simulink model "c00004M_harness"  (R2018a)
settings: Solver=FixedStepAuto  StartTime=0.0  StopTime=300  FixedStep=0.1  RelTol=1e-3
undefined symbols (not defined in the file): A1, hmax, R1, R2, sigbuilder_block, TempThreshold
(part 1 of 14)
settings Model: Creator=aarrieta  LastModifiedBy=umarkiegi

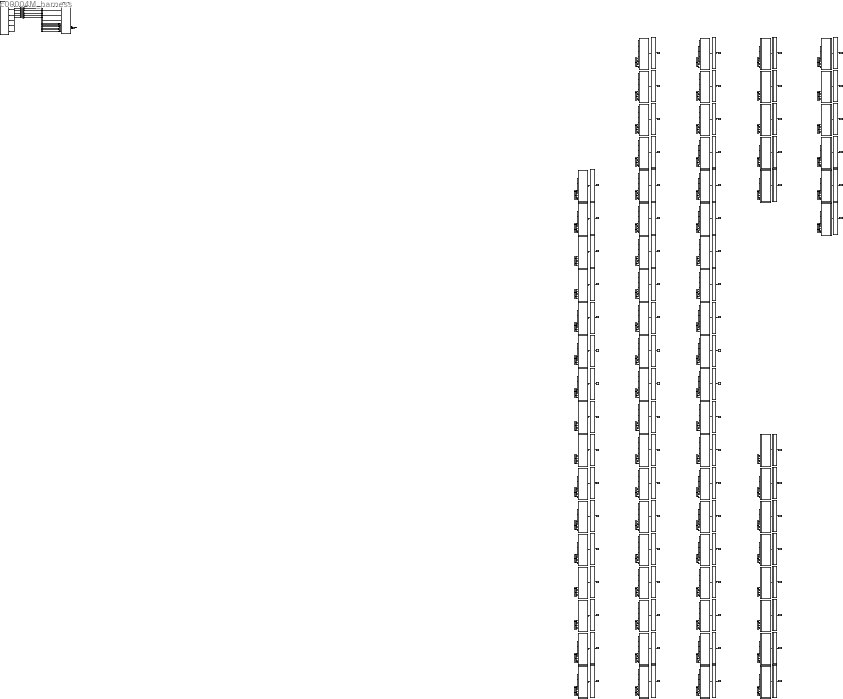
== system c00004M_harness ==
  CPSUT : Subsystem
  Eval164 : Subsystem
  Eval165 : Subsystem
  Eval166 : Subsystem
  Eval167 : Subsystem
  Eval168 : Subsystem
  Eval169 : Subsystem
  Eval170 : Subsystem
  Eval171 : Subsystem
  Eval172 : Subsystem
  Eval173 : Subsystem
  Eval174 : Subsystem
  Eval175 : Subsystem
  Eval176 : Subsystem
  Eval177 : Subsystem
  Eval178 : Subsystem
  Eval179 : Subsystem
  Eval180 : Subsystem
  Eval181 : Subsystem
  Eval182 : Subsystem
  Eval183 : Subsystem
  Eval184 : Subsystem
  Eval185 : Subsystem
  Eval186 : Subsystem
  Eval187 : Subsystem
  Eval188 : Subsystem
  Eval189 : Subsystem
  Eval190 : Subsystem
  Eval191 : Subsystem
  Eval192 : Subsystem
  Eval193 : Subsystem
  Eval194 : Subsystem
  Eval195 : Subsystem
  Eval196 : Subsystem
  Eval197 : Subsystem
  Eval198 : Subsystem
  Eval199 : Subsystem
  Eval200 : Subsystem
  Eval201 : Subsystem
  Eval202 : Subsystem
  Eval203 : Subsystem
  Eval204 : Subsystem
  Eval205 : Subsystem
  Eval206 : Subsystem
  Eval207 : Subsystem
  Eval208 : Subsystem
  Eval209 : Subsystem
  Eval210 : Subsystem
  Eval211 : Subsystem
  Eval212 : Subsystem
  Eval213 : Subsystem
  Eval214 : Subsystem
  Eval215 : Subsystem
  Eval216 : Subsystem
  Eval217 : Subsystem
  Eval218 : Subsystem
  Eval219 : Subsystem
  Eval220 : Subsystem
  Eval221 : Subsystem
  Eval222 : Subsystem
  Eval223 : Subsystem
  Eval224 : Subsystem
  Eval232 : Subsystem
  Eval233 : Subsystem
  Eval234 : Subsystem
  Eval235 : Subsystem
  Eval236 : Subsystem
  Eval237 : Subsystem
  Eval238 : Subsystem
  Eval239 : Subsystem
  Eval240 : Subsystem
  Eval241 : Subsystem
  Eval242 : Subsystem
  Eval243 : Subsystem
  Eval244 : Subsystem
  Eval245 : Subsystem
  Inputs : Subsystem  Tag=STV Subsys  LoadFcn=sigbuilder_block('load');  StartFcn=sigbuilder_block('start');  StopFcn=sigbuilder_block('stop');  ClipboardFcn=sigbuilder_block('clipboard');  mask(Sigbuilder block){tuvar=[0:10]}
      mask init:
      | if ~strcmp(get_param(bdroot(gcb),'SimulationStatus'),'stopped'),tuvar = sigbuilder_block('maskInit'); end
      settings: CopyFcn=sigbuilder_block('copy');  DeleteFcn=sigbuilder_block('delete');  ModelCloseFcn=sigbuilder_block('modelClose');  PreSaveFcn=sigbuilder_block('preSave');  PauseFcn=sigbuilder_block('pause');  ContinueFcn=sigbuilder_block('continue');  NameChangeFcn=sigbuilder_block('namechange');  OpenFcn=sigbuilder_block('open',[276.75 163.5 675.75 486.75 ]);  CloseFcn=sigbuilder_block('close');
      mask Display: plot(0, 0, 100, 100,[2, 2, 32, 32, 2], [68, 8, 8, 68, 68],[32, 2], [38, 38], [32, 19, 2],[53, 60, 44], [32, 17, 17, 2],[16, 16, 31, 31]);txt = getActiveGroup(gcbh);text(2, 100, txt,'verticalAlignment', 'top');
  M165 : Subsystem
  M166 : Subsystem
  M167 : Subsystem
  M168 : Subsystem
  M169 : Subsystem
  M170 : Subsystem
  M171 : Subsystem
  M172 : Subsystem
  M173 : Subsystem
  M174 : Subsystem
  M175 : Subsystem
  M176 : Subsystem
  M177 : Subsystem
  M178 : Subsystem
  M179 : Subsystem
  M180 : Subsystem
  M181 : Subsystem
  M182 : Subsystem
  M183 : Subsystem
  M184 : Subsystem
  M185 : Subsystem
  M186 : Subsystem
  M187 : Subsystem
  M188 : Subsystem
  M189 : Subsystem
  M190 : Subsystem
  M191 : Subsystem
  M192 : Subsystem
  M193 : Subsystem
  M194 : Subsystem
  M195 : Subsystem
  M196 : Subsystem
  M197 : Subsystem
  M198 : Subsystem
  M199 : Subsystem
  M200 : Subsystem
  M201 : Subsystem
  M202 : Subsystem
  M203 : Subsystem
  M204 : Subsystem
  M205 : Subsystem
  M206 : Subsystem
  M207 : Subsystem
  M208 : Subsystem
  M209 : Subsystem
  M210 : Subsystem
  M211 : Subsystem
  M212 : Subsystem
  M213 : Subsystem
  M214 : Subsystem
  M215 : Subsystem
  M216 : Subsystem
  M217 : Subsystem
  M218 : Subsystem
  M219 : Subsystem
  M220 : Subsystem
  M221 : Subsystem
  M222 : Subsystem
  M223 : Subsystem
  M224 : Subsystem
  M225 : Subsystem
  M233 : Subsystem
  M234 : Subsystem
  M235 : Subsystem
  M236 : Subsystem
  M237 : Subsystem
  M238 : Subsystem
  M239 : Subsystem
  M240 : Subsystem
  M241 : Subsystem
  M242 : Subsystem
  M243 : Subsystem
  M244 : Subsystem
  M245 : Subsystem
  M246 : Subsystem
  To Workspace164 : ToWorkspace  VariableName=mutant165  SampleTime=-1
  To Workspace165 : ToWorkspace  VariableName=mutant166  SampleTime=-1
  To Workspace166 : ToWorkspace  VariableName=mutant167  SampleTime=-1
  To Workspace167 : ToWorkspace  VariableName=mutant168  SampleTime=-1
  To Workspace168 : ToWorkspace  VariableName=mutant169  SampleTime=-1
  To Workspace169 : ToWorkspace  VariableName=mutant170  SampleTime=-1
  To Workspace170 : ToWorkspace  VariableName=mutant171  SampleTime=-1
  To Workspace171 : ToWorkspace  VariableName=mutant172  SampleTime=-1
  To Workspace172 : ToWorkspace  VariableName=mutant173  SampleTime=-1
  To Workspace173 : ToWorkspace  VariableName=mutant174  SampleTime=-1
  To Workspace174 : ToWorkspace  VariableName=mutant175  SampleTime=-1
  To Workspace175 : ToWorkspace  VariableName=mutant176  SampleTime=-1
  To Workspace176 : ToWorkspace  VariableName=mutant177  SampleTime=-1
  To Workspace177 : ToWorkspace  VariableName=mutant178  SampleTime=-1
  To Workspace178 : ToWorkspace  VariableName=mutant179  SampleTime=-1
  To Workspace179 : ToWorkspace  VariableName=mutant180  SampleTime=-1
  To Workspace180 : ToWorkspace  VariableName=mutant181  SampleTime=-1
  To Workspace181 : ToWorkspace  VariableName=mutant182  SampleTime=-1
  To Workspace182 : ToWorkspace  VariableName=mutant183  SampleTime=-1
  To Workspace183 : ToWorkspace  VariableName=mutant184  SampleTime=-1
  To Workspace184 : ToWorkspace  VariableName=mutant185  SampleTime=-1
  To Workspace185 : ToWorkspace  VariableName=mutant186  SampleTime=-1
  To Workspace186 : ToWorkspace  VariableName=mutant187  SampleTime=-1
  To Workspace187 : ToWorkspace  VariableName=mutant188  SampleTime=-1
  To Workspace188 : ToWorkspace  VariableName=mutant189  SampleTime=-1
  To Workspace189 : ToWorkspace  VariableName=mutant190  SampleTime=-1
  To Workspace190 : ToWorkspace  VariableName=mutant191  SampleTime=-1
  To Workspace191 : ToWorkspace  VariableName=mutant192  SampleTime=-1
  To Workspace192 : ToWorkspace  VariableName=mutant193  SampleTime=-1
  To Workspace193 : ToWorkspace  VariableName=mutant194  SampleTime=-1
  To Workspace194 : ToWorkspace  VariableName=mutant195  SampleTime=-1
  To Workspace195 : ToWorkspace  VariableName=mutant196  SampleTime=-1
  To Workspace196 : ToWorkspace  VariableName=mutant197  SampleTime=-1
  To Workspace197 : ToWorkspace  VariableName=mutant198  SampleTime=-1
  To Workspace198 : ToWorkspace  VariableName=mutant199  SampleTime=-1
  To Workspace199 : ToWorkspace  VariableName=mutant200  SampleTime=-1
  To Workspace200 : ToWorkspace  VariableName=mutant201  SampleTime=-1
  To Workspace201 : ToWorkspace  VariableName=mutant202  SampleTime=-1
  To Workspace202 : ToWorkspace  VariableName=mutant203  SampleTime=-1
  To Workspace203 : ToWorkspace  VariableName=mutant204  SampleTime=-1
  To Workspace204 : ToWorkspace  VariableName=mutant205  SampleTime=-1
  To Workspace205 : ToWorkspace  VariableName=mutant206  SampleTime=-1
  To Workspace206 : ToWorkspace  VariableName=mutant207  SampleTime=-1
  To Workspace207 : ToWorkspace  VariableName=mutant208  SampleTime=-1
  To Workspace208 : ToWorkspace  VariableName=mutant209  SampleTime=-1
  To Workspace209 : ToWorkspace  VariableName=mutant210  SampleTime=-1
  To Workspace210 : ToWorkspace  VariableName=mutant211  SampleTime=-1
  To Workspace211 : ToWorkspace  VariableName=mutant212  SampleTime=-1
  To Workspace212 : ToWorkspace  VariableName=mutant213  SampleTime=-1
  To Workspace213 : ToWorkspace  VariableName=mutant214  SampleTime=-1
  To Workspace214 : ToWorkspace  VariableName=mutant215  SampleTime=-1
  To Workspace215 : ToWorkspace  VariableName=mutant216  SampleTime=-1
  To Workspace216 : ToWorkspace  VariableName=mutant217  SampleTime=-1
  To Workspace217 : ToWorkspace  VariableName=mutant218  SampleTime=-1
  To Workspace218 : ToWorkspace  VariableName=mutant219  SampleTime=-1
  To Workspace219 : ToWorkspace  VariableName=mutant220  SampleTime=-1
  To Workspace220 : ToWorkspace  VariableName=mutant221  SampleTime=-1
  To Workspace221 : ToWorkspace  VariableName=mutant222  SampleTime=-1
  To Workspace222 : ToWorkspace  VariableName=mutant223  SampleTime=-1
  To Workspace223 : ToWorkspace  VariableName=mutant224  SampleTime=-1
  To Workspace224 : ToWorkspace  VariableName=mutant225  SampleTime=-1
  To Workspace232 : ToWorkspace  VariableName=mutant233  SampleTime=-1
  To Workspace233 : ToWorkspace  VariableName=mutant234  SampleTime=-1
  To Workspace234 : ToWorkspace  VariableName=mutant235  SampleTime=-1
  To Workspace235 : ToWorkspace  VariableName=mutant236  SampleTime=-1
  To Workspace236 : ToWorkspace  VariableName=mutant237  SampleTime=-1
  To Workspace237 : ToWorkspace  VariableName=mutant238  SampleTime=-1
  To Workspace238 : ToWorkspace  VariableName=mutant239  SampleTime=-1
  To Workspace239 : ToWorkspace  VariableName=mutant240  SampleTime=-1
  To Workspace240 : ToWorkspace  VariableName=mutant241  SampleTime=-1
  To Workspace241 : ToWorkspace  VariableName=mutant242  SampleTime=-1
  To Workspace242 : ToWorkspace  VariableName=mutant243  SampleTime=-1
  To Workspace243 : ToWorkspace  VariableName=mutant244  SampleTime=-1
  To Workspace244 : ToWorkspace  VariableName=mutant245  SampleTime=-1
  To Workspace245 : ToWorkspace  VariableName=mutant246  SampleTime=-1
  dtc_CT3 : DataTypeConversion
  dtc_E3 : DataTypeConversion
  dtc_EB3 : DataTypeConversion
  dtc_F3 : DataTypeConversion
  dtc_MR3 : DataTypeConversion
  dtc_T3 : DataTypeConversion
  LL3 : Outport
  tag scope: out3=global
  wires:
  CPSUT/1(LL3) -> [out3], LL3/1
  [in13] -> M165/1(CT3)
  [in14] -> M165/2(F3)
  [in15] -> M165/3(E3)
  [in16] -> M165/4(MR3)
  [in17] -> M165/5(T3)
  [in18] -> M165/6(EB3)
  M165/1(LL3) -> Eval164/1(In3)
  Eval164/1(Out1) -> To Workspace164/1
  [in13] -> M166/1(CT3)
  [in14] -> M166/2(F3)
  [in15] -> M166/3(E3)
  [in16] -> M166/4(MR3)
  [in17] -> M166/5(T3)
  [in18] -> M166/6(EB3)
  M166/1(LL3) -> Eval165/1(In3)
  Eval165/1(Out1) -> To Workspace165/1
  [in13] -> M167/1(CT3)
  [in14] -> M167/2(F3)
  [in15] -> M167/3(E3)
  [in16] -> M167/4(MR3)
  [in17] -> M167/5(T3)
  [in18] -> M167/6(EB3)
  M167/1(LL3) -> Eval166/1(In3)
  Eval166/1(Out1) -> To Workspace166/1
  [in13] -> M168/1(CT3)
  [in14] -> M168/2(F3)
  [in15] -> M168/3(E3)
  [in16] -> M168/4(MR3)
  [in17] -> M168/5(T3)
  [in18] -> M168/6(EB3)
  M168/1(LL3) -> Eval167/1(In3)
  Eval167/1(Out1) -> To Workspace167/1
  [in13] -> M169/1(CT3)
  [in14] -> M169/2(F3)
  [in15] -> M169/3(E3)
  [in16] -> M169/4(MR3)
  [in17] -> M169/5(T3)
  [in18] -> M169/6(EB3)
  M169/1(LL3) -> Eval168/1(In3)
  Eval168/1(Out1) -> To Workspace168/1
  [in13] -> M170/1(CT3)
  [in14] -> M170/2(F3)
  [in15] -> M170/3(E3)
  [in16] -> M170/4(MR3)
  [in17] -> M170/5(T3)
  [in18] -> M170/6(EB3)
  M170/1(LL3) -> Eval169/1(In3)
  Eval169/1(Out1) -> To Workspace169/1
  [in13] -> M171/1(CT3)
  [in14] -> M171/2(F3)
  [in15] -> M171/3(E3)
  [in16] -> M171/4(MR3)
  [in17] -> M171/5(T3)
  [in18] -> M171/6(EB3)
  M171/1(LL3) -> Eval170/1(In3)
  Eval170/1(Out1) -> To Workspace170/1
  [in13] -> M172/1(CT3)
  [in14] -> M172/2(F3)
  [in15] -> M172/3(E3)
  [in16] -> M172/4(MR3)
  [in17] -> M172/5(T3)
  [in18] -> M172/6(EB3)
  M172/1(LL3) -> Eval171/1(In3)
  Eval171/1(Out1) -> To Workspace171/1
  [in13] -> M173/1(CT3)
  [in14] -> M173/2(F3)
  [in15] -> M173/3(E3)
  [in16] -> M173/4(MR3)
  [in17] -> M173/5(T3)
  [in18] -> M173/6(EB3)
  M173/1(LL3) -> Eval172/1(In3)
  Eval172/1(Out1) -> To Workspace172/1
  [in13] -> M174/1(CT3)
  [in14] -> M174/2(F3)
  [in15] -> M174/3(E3)
  [in16] -> M174/4(MR3)
  [in17] -> M174/5(T3)
  [in18] -> M174/6(EB3)
  M174/1(LL3) -> Eval173/1(In3)
  Eval173/1(Out1) -> To Workspace173/1
  [in13] -> M175/1(CT3)
  [in14] -> M175/2(F3)
  [in15] -> M175/3(E3)
  [in16] -> M175/4(MR3)
  [in17] -> M175/5(T3)
  [in18] -> M175/6(EB3)
  M175/1(LL3) -> Eval174/1(In3)
  Eval174/1(Out1) -> To Workspace174/1
  [in13] -> M176/1(CT3)
  [in14] -> M176/2(F3)
  [in15] -> M176/3(E3)
  [in16] -> M176/4(MR3)
  [in17] -> M176/5(T3)
  [in18] -> M176/6(EB3)
  M176/1(LL3) -> Eval175/1(In3)
  Eval175/1(Out1) -> To Workspace175/1
  [in13] -> M177/1(CT3)
  [in14] -> M177/2(F3)
  [in15] -> M177/3(E3)
  [in16] -> M177/4(MR3)
  [in17] -> M177/5(T3)
  [in18] -> M177/6(EB3)
  M177/1(LL3) -> Eval176/1(In3)
  Eval176/1(Out1) -> To Workspace176/1
  [in13] -> M178/1(CT3)
  [in14] -> M178/2(F3)
  [in15] -> M178/3(E3)
  [in16] -> M178/4(MR3)
  [in17] -> M178/5(T3)
  [in18] -> M178/6(EB3)
  M178/1(LL3) -> Eval177/1(In3)
  Eval177/1(Out1) -> To Workspace177/1
  [in13] -> M179/1(CT3)
  [in14] -> M179/2(F3)
  [in15] -> M179/3(E3)
  [in16] -> M179/4(MR3)
  [in17] -> M179/5(T3)
  [in18] -> M179/6(EB3)
  M179/1(LL3) -> Eval178/1(In3)
  Eval178/1(Out1) -> To Workspace178/1
  [in13] -> M180/1(CT3)
  [in14] -> M180/2(F3)
  [in15] -> M180/3(E3)
  [in16] -> M180/4(MR3)
  [in17] -> M180/5(T3)
  [in18] -> M180/6(EB3)
  M180/1(LL3) -> Eval179/1(In3)
  Eval179/1(Out1) -> To Workspace179/1
  [in13] -> M181/1(CT3)
  [in14] -> M181/2(F3)
  [in15] -> M181/3(E3)
  [in16] -> M181/4(MR3)
  [in17] -> M181/5(T3)
  [in18] -> M181/6(EB3)
  M181/1(LL3) -> Eval180/1(In3)
  Eval180/1(Out1) -> To Workspace180/1
  [in13] -> M182/1(CT3)
  [in14] -> M182/2(F3)
  [in15] -> M182/3(E3)
  [in16] -> M182/4(MR3)
  [in17] -> M182/5(T3)
  [in18] -> M182/6(EB3)
  M182/1(LL3) -> Eval181/1(In3)
  Eval181/1(Out1) -> To Workspace181/1
  [in13] -> M183/1(CT3)
  [in14] -> M183/2(F3)
  [in15] -> M183/3(E3)
  [in16] -> M183/4(MR3)
  [in17] -> M183/5(T3)
  [in18] -> M183/6(EB3)
  M183/1(LL3) -> Eval182/1(In3)
  Eval182/1(Out1) -> To Workspace182/1
  [in13] -> M184/1(CT3)
  [in14] -> M184/2(F3)
  [in15] -> M184/3(E3)
  [in16] -> M184/4(MR3)
  [in17] -> M184/5(T3)
  [in18] -> M184/6(EB3)
  M184/1(LL3) -> Eval183/1(In3)
  Eval183/1(Out1) -> To Workspace183/1
  [in13] -> M185/1(CT3)
  [in14] -> M185/2(F3)
  [in15] -> M185/3(E3)
  [in16] -> M185/4(MR3)
  [in17] -> M185/5(T3)
  [in18] -> M185/6(EB3)
  M185/1(LL3) -> Eval184/1(In3)
  Eval184/1(Out1) -> To Workspace184/1
  [in13] -> M186/1(CT3)
  [in14] -> M186/2(F3)
  [in15] -> M186/3(E3)
  [in16] -> M186/4(MR3)
  [in17] -> M186/5(T3)
  [in18] -> M186/6(EB3)
  M186/1(LL3) -> Eval185/1(In3)
  Eval185/1(Out1) -> To Workspace185/1
  [in13] -> M187/1(CT3)
  [in14] -> M187/2(F3)
  [in15] -> M187/3(E3)
  [in16] -> M187/4(MR3)
  [in17] -> M187/5(T3)
  [in18] -> M187/6(EB3)
  M187/1(LL3) -> Eval186/1(In3)
  Eval186/1(Out1) -> To Workspace186/1
  [in13] -> M188/1(CT3)
  [in14] -> M188/2(F3)
  [in15] -> M188/3(E3)
  [in16] -> M188/4(MR3)
  [in17] -> M188/5(T3)
  [in18] -> M188/6(EB3)
  M188/1(LL3) -> Eval187/1(In3)
  Eval187/1(Out1) -> To Workspace187/1
  [in13] -> M189/1(CT3)
  [in14] -> M189/2(F3)
  [in15] -> M189/3(E3)
  [in16] -> M189/4(MR3)
  [in17] -> M189/5(T3)
  [in18] -> M189/6(EB3)
  M189/1(LL3) -> Eval188/1(In3)
  Eval188/1(Out1) -> To Workspace188/1
  [in13] -> M190/1(CT3)
  [in14] -> M190/2(F3)
  [in15] -> M190/3(E3)
  [in16] -> M190/4(MR3)
  [in17] -> M190/5(T3)
  [in18] -> M190/6(EB3)
  M190/1(LL3) -> Eval189/1(In3)
  Eval189/1(Out1) -> To Workspace189/1
  [in13] -> M191/1(CT3)
  [in14] -> M191/2(F3)
  [in15] -> M191/3(E3)
  [in16] -> M191/4(MR3)
  [in17] -> M191/5(T3)
  [in18] -> M191/6(EB3)
  M191/1(LL3) -> Eval190/1(In3)
  Eval190/1(Out1) -> To Workspace190/1
  [in13] -> M192/1(CT3)
  [in14] -> M192/2(F3)
  [in15] -> M192/3(E3)
  [in16] -> M192/4(MR3)
  [in17] -> M192/5(T3)
  [in18] -> M192/6(EB3)
  M192/1(LL3) -> Eval191/1(In3)
  Eval191/1(Out1) -> To Workspace191/1
  [in13] -> M193/1(CT3)
  [in14] -> M193/2(F3)
  [in15] -> M193/3(E3)
  [in16] -> M193/4(MR3)
  [in17] -> M193/5(T3)
  [in18] -> M193/6(EB3)
  M193/1(LL3) -> Eval192/1(In3)
  Eval192/1(Out1) -> To Workspace192/1
  [in13] -> M194/1(CT3)
  [in14] -> M194/2(F3)
  [in15] -> M194/3(E3)
  [in16] -> M194/4(MR3)
  [in17] -> M194/5(T3)
  [in18] -> M194/6(EB3)
  M194/1(LL3) -> Eval193/1(In3)
  Eval193/1(Out1) -> To Workspace193/1
  [in13] -> M195/1(CT3)
  [in14] -> M195/2(F3)
  [in15] -> M195/3(E3)
  [in16] -> M195/4(MR3)
  [in17] -> M195/5(T3)
  [in18] -> M195/6(EB3)
  M195/1(LL3) -> Eval194/1(In3)
  Eval194/1(Out1) -> To Workspace194/1
  [in13] -> M196/1(CT3)
  [in14] -> M196/2(F3)
  [in15] -> M196/3(E3)
  [in16] -> M196/4(MR3)
  [in17] -> M196/5(T3)
  [in18] -> M196/6(EB3)
  M196/1(LL3) -> Eval195/1(In3)
  Eval195/1(Out1) -> To Workspace195/1
  [in13] -> M197/1(CT3)
  [in14] -> M197/2(F3)
  [in15] -> M197/3(E3)
  [in16] -> M197/4(MR3)
  [in17] -> M197/5(T3)
  [in18] -> M197/6(EB3)
  M197/1(LL3) -> Eval196/1(In3)
  Eval196/1(Out1) -> To Workspace196/1
  [in13] -> M198/1(CT3)
  [in14] -> M198/2(F3)
  [in15] -> M198/3(E3)
  [in16] -> M198/4(MR3)
  [in17] -> M198/5(T3)
  [in18] -> M198/6(EB3)
  M198/1(LL3) -> Eval197/1(In3)
  Eval197/1(Out1) -> To Workspace197/1
  [in13] -> M199/1(CT3)
  [in14] -> M199/2(F3)
  [in15] -> M199/3(E3)
  [in16] -> M199/4(MR3)
  [in17] -> M199/5(T3)
  [in18] -> M199/6(EB3)
  M199/1(LL3) -> Eval198/1(In3)
  Eval198/1(Out1) -> To Workspace198/1
  [in13] -> M200/1(CT3)
  [in14] -> M200/2(F3)
  [in15] -> M200/3(E3)
  [in16] -> M200/4(MR3)
  [in17] -> M200/5(T3)
  [in18] -> M200/6(EB3)
  M200/1(LL3) -> Eval199/1(In3)
  Eval199/1(Out1) -> To Workspace199/1
  [in13] -> M201/1(CT3)
  [in14] -> M201/2(F3)
  [in15] -> M201/3(E3)
  [in16] -> M201/4(MR3)
  [in17] -> M201/5(T3)
  [in18] -> M201/6(EB3)
  M201/1(LL3) -> Eval200/1(In3)
  Eval200/1(Out1) -> To Workspace200/1
  [in13] -> M202/1(CT3)
  [in14] -> M202/2(F3)
  [in15] -> M202/3(E3)
  [in16] -> M202/4(MR3)
  [in17] -> M202/5(T3)
  [in18] -> M202/6(EB3)
  M202/1(LL3) -> Eval201/1(In3)
  Eval201/1(Out1) -> To Workspace201/1
  [in13] -> M203/1(CT3)
  [in14] -> M203/2(F3)
  [in15] -> M203/3(E3)
  [in16] -> M203/4(MR3)
  [in17] -> M203/5(T3)
  [in18] -> M203/6(EB3)
  M203/1(LL3) -> Eval202/1(In3)
  Eval202/1(Out1) -> To Workspace202/1
  [in13] -> M204/1(CT3)
  [in14] -> M204/2(F3)
  [in15] -> M204/3(E3)
  [in16] -> M204/4(MR3)
  [in17] -> M204/5(T3)
  [in18] -> M204/6(EB3)
  M204/1(LL3) -> Eval203/1(In3)
  Eval203/1(Out1) -> To Workspace203/1
  [in13] -> M205/1(CT3)
  [in14] -> M205/2(F3)
  [in15] -> M205/3(E3)
  [in16] -> M205/4(MR3)
  [in17] -> M205/5(T3)
  [in18] -> M205/6(EB3)
  M205/1(LL3) -> Eval204/1(In3)
  Eval204/1(Out1) -> To Workspace204/1
  [in13] -> M206/1(CT3)
  [in14] -> M206/2(F3)
  [in15] -> M206/3(E3)
  [in16] -> M206/4(MR3)
  [in17] -> M206/5(T3)
  [in18] -> M206/6(EB3)
  M206/1(LL3) -> Eval205/1(In3)
  Eval205/1(Out1) -> To Workspace205/1
  [in13] -> M207/1(CT3)
  [in14] -> M207/2(F3)
  [in15] -> M207/3(E3)
  [in16] -> M207/4(MR3)
  [in17] -> M207/5(T3)
  [in18] -> M207/6(EB3)
  M207/1(LL3) -> Eval206/1(In3)
  Eval206/1(Out1) -> To Workspace206/1
  [in13] -> M208/1(CT3)
  [in14] -> M208/2(F3)
  [in15] -> M208/3(E3)
  [in16] -> M208/4(MR3)
  [in17] -> M208/5(T3)
  [in18] -> M208/6(EB3)
  M208/1(LL3) -> Eval207/1(In3)
  Eval207/1(Out1) -> To Workspace207/1
  [in13] -> M209/1(CT3)
  [in14] -> M209/2(F3)
  [in15] -> M209/3(E3)
  [in16] -> M209/4(MR3)
  [in17] -> M209/5(T3)
  [in18] -> M209/6(EB3)
  M209/1(LL3) -> Eval208/1(In3)
  Eval208/1(Out1) -> To Workspace208/1
  [in13] -> M210/1(CT3)
  [in14] -> M210/2(F3)
  [in15] -> M210/3(E3)
  [in16] -> M210/4(MR3)
  [in17] -> M210/5(T3)
  [in18] -> M210/6(EB3)
  M210/1(LL3) -> Eval209/1(In3)
  Eval209/1(Out1) -> To Workspace209/1
  [in13] -> M211/1(CT3)
  [in14] -> M211/2(F3)
  [in15] -> M211/3(E3)
  [in16] -> M211/4(MR3)
  [in17] -> M211/5(T3)
  [in18] -> M211/6(EB3)
  M211/1(LL3) -> Eval210/1(In3)
  Eval210/1(Out1) -> To Workspace210/1
  [in13] -> M212/1(CT3)
  [in14] -> M212/2(F3)
  [in15] -> M212/3(E3)
  [in16] -> M212/4(MR3)
  [in17] -> M212/5(T3)
  [in18] -> M212/6(EB3)
  M212/1(LL3) -> Eval211/1(In3)
  Eval211/1(Out1) -> To Workspace211/1
  [in13] -> M213/1(CT3)
  [in14] -> M213/2(F3)
  [in15] -> M213/3(E3)
  [in16] -> M213/4(MR3)
  [in17] -> M213/5(T3)
  [in18] -> M213/6(EB3)
  M213/1(LL3) -> Eval212/1(In3)
  Eval212/1(Out1) -> To Workspace212/1
  [in13] -> M214/1(CT3)
  [in14] -> M214/2(F3)
  [in15] -> M214/3(E3)
  [in16] -> M214/4(MR3)
  [in17] -> M214/5(T3)
  [in18] -> M214/6(EB3)
  M214/1(LL3) -> Eval213/1(In3)
  Eval213/1(Out1) -> To Workspace213/1
  [in13] -> M215/1(CT3)
  [in14] -> M215/2(F3)
  [in15] -> M215/3(E3)
  [in16] -> M215/4(MR3)
  [in17] -> M215/5(T3)
  [in18] -> M215/6(EB3)
  M215/1(LL3) -> Eval214/1(In3)
  Eval214/1(Out1) -> To Workspace214/1
  [in13] -> M216/1(CT3)
  [in14] -> M216/2(F3)
  [in15] -> M216/3(E3)
  [in16] -> M216/4(MR3)
  [in17] -> M216/5(T3)
  [in18] -> M216/6(EB3)
  M216/1(LL3) -> Eval215/1(In3)
  Eval215/1(Out1) -> To Workspace215/1
  [in13] -> M217/1(CT3)
  [in14] -> M217/2(F3)
  [in15] -> M217/3(E3)
  [in16] -> M217/4(MR3)
  [in17] -> M217/5(T3)
  [in18] -> M217/6(EB3)
  M217/1(LL3) -> Eval216/1(In3)
  Eval216/1(Out1) -> To Workspace216/1
  [in13] -> M218/1(CT3)
  [in14] -> M218/2(F3)
  [in15] -> M218/3(E3)
  [in16] -> M218/4(MR3)
  [in17] -> M218/5(T3)
  [in18] -> M218/6(EB3)
  M218/1(LL3) -> Eval217/1(In3)
  Eval217/1(Out1) -> To Workspace217/1
  [in13] -> M219/1(CT3)
  [in14] -> M219/2(F3)
  [in15] -> M219/3(E3)
  [in16] -> M219/4(MR3)
  [in17] -> M219/5(T3)
  [in18] -> M219/6(EB3)
  M219/1(LL3) -> Eval218/1(In3)
  Eval218/1(Out1) -> To Workspace218/1
  [in13] -> M220/1(CT3)
  [in14] -> M220/2(F3)
  [in15] -> M220/3(E3)
  [in16] -> M220/4(MR3)
  [in17] -> M220/5(T3)
  [in18] -> M220/6(EB3)
  M220/1(LL3) -> Eval219/1(In3)
  Eval219/1(Out1) -> To Workspace219/1
  [in13] -> M221/1(CT3)
  [in14] -> M221/2(F3)
  [in15] -> M221/3(E3)
  [in16] -> M221/4(MR3)
  [in17] -> M221/5(T3)
  [in18] -> M221/6(EB3)
  M221/1(LL3) -> Eval220/1(In3)
  Eval220/1(Out1) -> To Workspace220/1
  [in13] -> M222/1(CT3)
  [in14] -> M222/2(F3)
  [in15] -> M222/3(E3)
  [in16] -> M222/4(MR3)
  [in17] -> M222/5(T3)
  [in18] -> M222/6(EB3)
  M222/1(LL3) -> Eval221/1(In3)
  Eval221/1(Out1) -> To Workspace221/1
  [in13] -> M223/1(CT3)
  [in14] -> M223/2(F3)
  [in15] -> M223/3(E3)
  [in16] -> M223/4(MR3)
  [in17] -> M223/5(T3)
  [in18] -> M223/6(EB3)
  M223/1(LL3) -> Eval222/1(In3)
  Eval222/1(Out1) -> To Workspace222/1
  [in13] -> M224/1(CT3)
  [in14] -> M224/2(F3)
  [in15] -> M224/3(E3)
  [in16] -> M224/4(MR3)
  [in17] -> M224/5(T3)
  [in18] -> M224/6(EB3)
  M224/1(LL3) -> Eval223/1(In3)
  Eval223/1(Out1) -> To Workspace223/1
  [in13] -> M225/1(CT3)
  [in14] -> M225/2(F3)
  [in15] -> M225/3(E3)
  [in16] -> M225/4(MR3)
  [in17] -> M225/5(T3)
  [in18] -> M225/6(EB3)
  M225/1(LL3) -> Eval224/1(In3)
  Eval224/1(Out1) -> To Workspace224/1
  [in13] -> M233/1(CT3)
  [in14] -> M233/2(F3)
  [in15] -> M233/3(E3)
  [in16] -> M233/4(MR3)
  [in17] -> M233/5(T3)
  [in18] -> M233/6(EB3)
  M233/1(LL3) -> Eval232/1(In3)
  Eval232/1(Out1) -> To Workspace232/1
  [in13] -> M234/1(CT3)
  [in14] -> M234/2(F3)
  [in15] -> M234/3(E3)
  [in16] -> M234/4(MR3)
  [in17] -> M234/5(T3)
  [in18] -> M234/6(EB3)
  M234/1(LL3) -> Eval233/1(In3)
  Eval233/1(Out1) -> To Workspace233/1
  [in13] -> M235/1(CT3)
  [in14] -> M235/2(F3)
  [in15] -> M235/3(E3)
  [in16] -> M235/4(MR3)
  [in17] -> M235/5(T3)
  [in18] -> M235/6(EB3)
  M235/1(LL3) -> Eval234/1(In3)
  Eval234/1(Out1) -> To Workspace234/1
  [in13] -> M236/1(CT3)
  [in14] -> M236/2(F3)
  [in15] -> M236/3(E3)
  [in16] -> M236/4(MR3)
  [in17] -> M236/5(T3)
  [in18] -> M236/6(EB3)
  M236/1(LL3) -> Eval235/1(In3)
  Eval235/1(Out1) -> To Workspace235/1
  [in13] -> M237/1(CT3)
  [in14] -> M237/2(F3)
  [in15] -> M237/3(E3)
  [in16] -> M237/4(MR3)
  [in17] -> M237/5(T3)
  [in18] -> M237/6(EB3)
  M237/1(LL3) -> Eval236/1(In3)
  Eval236/1(Out1) -> To Workspace236/1
  [in13] -> M238/1(CT3)
  [in14] -> M238/2(F3)
  [in15] -> M238/3(E3)
  [in16] -> M238/4(MR3)
  [in17] -> M238/5(T3)
  [in18] -> M238/6(EB3)
  M238/1(LL3) -> Eval237/1(In3)
  Eval237/1(Out1) -> To Workspace237/1
  [in13] -> M239/1(CT3)
  [in14] -> M239/2(F3)
  [in15] -> M239/3(E3)
  [in16] -> M239/4(MR3)
  [in17] -> M239/5(T3)
  [in18] -> M239/6(EB3)
  M239/1(LL3) -> Eval238/1(In3)
  Eval238/1(Out1) -> To Workspace238/1
  [in13] -> M240/1(CT3)
  [in14] -> M240/2(F3)
  [in15] -> M240/3(E3)
  [in16] -> M240/4(MR3)
  [in17] -> M240/5(T3)
  [in18] -> M240/6(EB3)
  M240/1(LL3) -> Eval239/1(In3)
  Eval239/1(Out1) -> To Workspace239/1
  [in13] -> M241/1(CT3)
  [in14] -> M241/2(F3)
  [in15] -> M241/3(E3)
  [in16] -> M241/4(MR3)
  [in17] -> M241/5(T3)
  [in18] -> M241/6(EB3)
  M241/1(LL3) -> Eval240/1(In3)
  Eval240/1(Out1) -> To Workspace240/1
  [in13] -> M242/1(CT3)
  [in14] -> M242/2(F3)
  [in15] -> M242/3(E3)
  [in16] -> M242/4(MR3)
  [in17] -> M242/5(T3)
  [in18] -> M242/6(EB3)
  M242/1(LL3) -> Eval241/1(In3)
  Eval241/1(Out1) -> To Workspace241/1
  [in13] -> M243/1(CT3)
  [in14] -> M243/2(F3)
  [in15] -> M243/3(E3)
  [in16] -> M243/4(MR3)
  [in17] -> M243/5(T3)
  [in18] -> M243/6(EB3)
  M243/1(LL3) -> Eval242/1(In3)
  Eval242/1(Out1) -> To Workspace242/1
  [in13] -> M244/1(CT3)
  [in14] -> M244/2(F3)
  [in15] -> M244/3(E3)
  [in16] -> M244/4(MR3)
  [in17] -> M244/5(T3)
  [in18] -> M244/6(EB3)
  M244/1(LL3) -> Eval243/1(In3)
  Eval243/1(Out1) -> To Workspace243/1
  [in13] -> M245/1(CT3)
  [in14] -> M245/2(F3)
  [in15] -> M245/3(E3)
  [in16] -> M245/4(MR3)
  [in17] -> M245/5(T3)
  [in18] -> M245/6(EB3)
  M245/1(LL3) -> Eval244/1(In3)
  Eval244/1(Out1) -> To Workspace244/1
  [in13] -> M246/1(CT3)
  [in14] -> M246/2(F3)
  [in15] -> M246/3(E3)
  [in16] -> M246/4(MR3)
  [in17] -> M246/5(T3)
  [in18] -> M246/6(EB3)
  M246/1(LL3) -> Eval245/1(In3)
  Eval245/1(Out1) -> To Workspace245/1
  Inputs/1(CT3) -> dtc_CT3/1
  dtc_CT3/1 -> CPSUT/1(CT3), [in13]
  Inputs/2(F3) -> dtc_F3/1
  dtc_F3/1 -> CPSUT/2(F3), [in14]
  Inputs/3(E3) -> dtc_E3/1
  dtc_E3/1 -> CPSUT/3(E3), [in15]
  Inputs/4(MR3) -> dtc_MR3/1
  dtc_MR3/1 -> CPSUT/4(MR3), [in16]
  Inputs/5(T3) -> dtc_T3/1
  dtc_T3/1 -> CPSUT/5(T3), [in17]
  Inputs/6(EB3) -> dtc_EB3/1
  dtc_EB3/1 -> CPSUT/6(EB3), [in18]

== system c00004M_harness/CPSUT ==
  note: VALUES
      | ---------------------------------
      | ControlType = 1 | 2 | 3
      | FillTank = 0 | 1
      | EmptyTank = 0 | 1
      | ManualReference between 0 and 1
      | Tempreature between 0 and 100
      | EmergencyButton = 0 | 1
      | LiquidLevel between 0 and 1 (hmax)
  note: Inputs For Tank2
  note: NAMES
      | --------------------------------------------
      | CT1 = ControlType Tank 1
      | F1 = Fill Tank 1
      | E1 = Empty Tank 1
      | MR1 = Manual Reference Tank1
      | T1 = Temperature Tank 1
      | EB1 = Emergency Button Tank 1
      | LL1 = Liquid Level 1
  note: Inputs For Tank3
  note: Inputs For Tank1
  CT3 : Inport
  F3 : Inport  Port=2
  E3 : Inport  Port=3
  MR3 : Inport  Port=4
  T3 : Inport  Port=5
  EB3 : Inport  Port=6
  Tank3 : Subsystem
  LL3 : Outport
  wires:
  Tank3/1(LL3) -> LL3/1
  MR3/1 -> Tank3/4(MR3)
  E3/1 -> Tank3/3(E3)
  CT3/1 -> Tank3/1(CT3)
  F3/1 -> Tank3/2(F3)
  EB3/1 -> Tank3/6(EB3)
  T3/1 -> Tank3/5(T3)

== system c00004M_harness/Eval164 ==
  In3 : Inport
  Constant1 : Constant
  Constant2 : Constant
  Data Type Conversion2 : DataTypeConversion
  Memory3 : Memory  InitialCondition=1
  MinMax : MinMax  Inputs=3
  MinMax3 : MinMax  Inputs=2
  ROOut3 : RelationalOperator  Operator===  OutDataTypeStr=boolean  RndMeth=Simplest
  Out1 : Outport
  wires:
  Data Type Conversion2/1 -> MinMax3/1
  Memory3/1 -> MinMax3/2
  ROOut3/1 -> Data Type Conversion2/1
  MinMax3/1 -> Memory3/1, MinMax/3
  In3/1 -> ROOut3/1
  [out3] -> ROOut3/2
  MinMax/1 -> Out1/1
  Constant1/1 -> MinMax/1
  Constant2/1 -> MinMax/2

== system c00004M_harness/Eval165 ==
  In3 : Inport
  Constant1 : Constant
  Constant2 : Constant
  Data Type Conversion2 : DataTypeConversion
  Memory3 : Memory  InitialCondition=1
  MinMax : MinMax  Inputs=3
  MinMax3 : MinMax  Inputs=2
  ROOut3 : RelationalOperator  Operator===  OutDataTypeStr=boolean  RndMeth=Simplest
  Out1 : Outport
  wires:
  Data Type Conversion2/1 -> MinMax3/1
  Memory3/1 -> MinMax3/2
  ROOut3/1 -> Data Type Conversion2/1
  MinMax3/1 -> Memory3/1, MinMax/3
  In3/1 -> ROOut3/1
  [out3] -> ROOut3/2
  MinMax/1 -> Out1/1
  Constant1/1 -> MinMax/1
  Constant2/1 -> MinMax/2

== system c00004M_harness/Eval166 ==
  In3 : Inport
  Constant1 : Constant
  Constant2 : Constant
  Data Type Conversion2 : DataTypeConversion
  Memory3 : Memory  InitialCondition=1
  MinMax : MinMax  Inputs=3
  MinMax3 : MinMax  Inputs=2
  ROOut3 : RelationalOperator  Operator===  OutDataTypeStr=boolean  RndMeth=Simplest
  Out1 : Outport
  wires:
  Data Type Conversion2/1 -> MinMax3/1
  Memory3/1 -> MinMax3/2
  ROOut3/1 -> Data Type Conversion2/1
  MinMax3/1 -> Memory3/1, MinMax/3
  In3/1 -> ROOut3/1
  [out3] -> ROOut3/2
  MinMax/1 -> Out1/1
  Constant1/1 -> MinMax/1
  Constant2/1 -> MinMax/2

== system c00004M_harness/Eval167 ==
  In3 : Inport
  Constant1 : Constant
  Constant2 : Constant
  Data Type Conversion2 : DataTypeConversion
  Memory3 : Memory  InitialCondition=1
  MinMax : MinMax  Inputs=3
  MinMax3 : MinMax  Inputs=2
  ROOut3 : RelationalOperator  Operator===  OutDataTypeStr=boolean  RndMeth=Simplest
  Out1 : Outport
  wires:
  Data Type Conversion2/1 -> MinMax3/1
  Memory3/1 -> MinMax3/2
  ROOut3/1 -> Data Type Conversion2/1
  MinMax3/1 -> Memory3/1, MinMax/3
  In3/1 -> ROOut3/1
  [out3] -> ROOut3/2
  MinMax/1 -> Out1/1
  Constant1/1 -> MinMax/1
  Constant2/1 -> MinMax/2

== system c00004M_harness/Eval168 ==
  In3 : Inport
  Constant1 : Constant
  Constant2 : Constant
  Data Type Conversion2 : DataTypeConversion
  Memory3 : Memory  InitialCondition=1
  MinMax : MinMax  Inputs=3
  MinMax3 : MinMax  Inputs=2
  ROOut3 : RelationalOperator  Operator===  OutDataTypeStr=boolean  RndMeth=Simplest
  Out1 : Outport
  wires:
  Data Type Conversion2/1 -> MinMax3/1
  Memory3/1 -> MinMax3/2
  ROOut3/1 -> Data Type Conversion2/1
  MinMax3/1 -> Memory3/1, MinMax/3
  In3/1 -> ROOut3/1
  [out3] -> ROOut3/2
  MinMax/1 -> Out1/1
  Constant1/1 -> MinMax/1
  Constant2/1 -> MinMax/2

== system c00004M_harness/Eval169 ==
  In3 : Inport
  Constant1 : Constant
  Constant2 : Constant
  Data Type Conversion2 : DataTypeConversion
  Memory3 : Memory  InitialCondition=1
  MinMax : MinMax  Inputs=3
  MinMax3 : MinMax  Inputs=2
  ROOut3 : RelationalOperator  Operator===  OutDataTypeStr=boolean  RndMeth=Simplest
  Out1 : Outport
  wires:
  Data Type Conversion2/1 -> MinMax3/1
  Memory3/1 -> MinMax3/2
  ROOut3/1 -> Data Type Conversion2/1
  MinMax3/1 -> Memory3/1, MinMax/3
  In3/1 -> ROOut3/1
  [out3] -> ROOut3/2
  MinMax/1 -> Out1/1
  Constant1/1 -> MinMax/1
  Constant2/1 -> MinMax/2

== system c00004M_harness/Eval170 ==
  In3 : Inport
  Constant1 : Constant
  Constant2 : Constant
  Data Type Conversion2 : DataTypeConversion
  Memory3 : Memory  InitialCondition=1
  MinMax : MinMax  Inputs=3
  MinMax3 : MinMax  Inputs=2
  ROOut3 : RelationalOperator  Operator===  OutDataTypeStr=boolean  RndMeth=Simplest
  Out1 : Outport
  wires:
  Data Type Conversion2/1 -> MinMax3/1
  Memory3/1 -> MinMax3/2
  ROOut3/1 -> Data Type Conversion2/1
  MinMax3/1 -> Memory3/1, MinMax/3
  In3/1 -> ROOut3/1
  [out3] -> ROOut3/2
  MinMax/1 -> Out1/1
  Constant1/1 -> MinMax/1
  Constant2/1 -> MinMax/2

== system c00004M_harness/Eval171 ==
  In3 : Inport
  Constant1 : Constant
  Constant2 : Constant
  Data Type Conversion2 : DataTypeConversion
  Memory3 : Memory  InitialCondition=1
  MinMax : MinMax  Inputs=3
  MinMax3 : MinMax  Inputs=2
  ROOut3 : RelationalOperator  Operator===  OutDataTypeStr=boolean  RndMeth=Simplest
  Out1 : Outport
  wires:
  Data Type Conversion2/1 -> MinMax3/1
  Memory3/1 -> MinMax3/2
  ROOut3/1 -> Data Type Conversion2/1
  MinMax3/1 -> Memory3/1, MinMax/3
  In3/1 -> ROOut3/1
  [out3] -> ROOut3/2
  MinMax/1 -> Out1/1
  Constant1/1 -> MinMax/1
  Constant2/1 -> MinMax/2

== system c00004M_harness/Eval172 ==
  In3 : Inport
  Constant1 : Constant
  Constant2 : Constant
  Data Type Conversion2 : DataTypeConversion
  Memory3 : Memory  InitialCondition=1
  MinMax : MinMax  Inputs=3
  MinMax3 : MinMax  Inputs=2
  ROOut3 : RelationalOperator  Operator===  OutDataTypeStr=boolean  RndMeth=Simplest
  Out1 : Outport
  wires:
  Data Type Conversion2/1 -> MinMax3/1
  Memory3/1 -> MinMax3/2
  ROOut3/1 -> Data Type Conversion2/1
  MinMax3/1 -> Memory3/1, MinMax/3
  In3/1 -> ROOut3/1
  [out3] -> ROOut3/2
  MinMax/1 -> Out1/1
  Constant1/1 -> MinMax/1
  Constant2/1 -> MinMax/2

== system c00004M_harness/Eval173 ==
  In3 : Inport
  Constant1 : Constant
  Constant2 : Constant
  Data Type Conversion2 : DataTypeConversion
  Memory3 : Memory  InitialCondition=1
  MinMax : MinMax  Inputs=3
  MinMax3 : MinMax  Inputs=2
  ROOut3 : RelationalOperator  Operator===  OutDataTypeStr=boolean  RndMeth=Simplest
  Out1 : Outport
  wires:
  Data Type Conversion2/1 -> MinMax3/1
  Memory3/1 -> MinMax3/2
  ROOut3/1 -> Data Type Conversion2/1
  MinMax3/1 -> Memory3/1, MinMax/3
  In3/1 -> ROOut3/1
  [out3] -> ROOut3/2
  MinMax/1 -> Out1/1
  Constant1/1 -> MinMax/1
  Constant2/1 -> MinMax/2

== system c00004M_harness/Eval174 ==
  In3 : Inport
  Constant1 : Constant
  Constant2 : Constant
  Data Type Conversion2 : DataTypeConversion
  Memory3 : Memory  InitialCondition=1
  MinMax : MinMax  Inputs=3
  MinMax3 : MinMax  Inputs=2
  ROOut3 : RelationalOperator  Operator===  OutDataTypeStr=boolean  RndMeth=Simplest
  Out1 : Outport
  wires:
  Data Type Conversion2/1 -> MinMax3/1
  Memory3/1 -> MinMax3/2
  ROOut3/1 -> Data Type Conversion2/1
  MinMax3/1 -> Memory3/1, MinMax/3
  In3/1 -> ROOut3/1
  [out3] -> ROOut3/2
  MinMax/1 -> Out1/1
  Constant1/1 -> MinMax/1
  Constant2/1 -> MinMax/2

== system c00004M_harness/Eval175 ==
  In3 : Inport
  Constant1 : Constant
  Constant2 : Constant
  Data Type Conversion2 : DataTypeConversion
  Memory3 : Memory  InitialCondition=1
  MinMax : MinMax  Inputs=3
  MinMax3 : MinMax  Inputs=2
  ROOut3 : RelationalOperator  Operator===  OutDataTypeStr=boolean  RndMeth=Simplest
  Out1 : Outport
  wires:
  Data Type Conversion2/1 -> MinMax3/1
  Memory3/1 -> MinMax3/2
  ROOut3/1 -> Data Type Conversion2/1
  MinMax3/1 -> Memory3/1, MinMax/3
  In3/1 -> ROOut3/1
  [out3] -> ROOut3/2
  MinMax/1 -> Out1/1
  Constant1/1 -> MinMax/1
  Constant2/1 -> MinMax/2

== system c00004M_harness/Eval176 ==
  In3 : Inport
  Constant1 : Constant
  Constant2 : Constant
  Data Type Conversion2 : DataTypeConversion
  Memory3 : Memory  InitialCondition=1
  MinMax : MinMax  Inputs=3
  MinMax3 : MinMax  Inputs=2
  ROOut3 : RelationalOperator  Operator===  OutDataTypeStr=boolean  RndMeth=Simplest
  Out1 : Outport
  wires:
  Data Type Conversion2/1 -> MinMax3/1
  Memory3/1 -> MinMax3/2
  ROOut3/1 -> Data Type Conversion2/1
  MinMax3/1 -> Memory3/1, MinMax/3
  In3/1 -> ROOut3/1
  [out3] -> ROOut3/2
  MinMax/1 -> Out1/1
  Constant1/1 -> MinMax/1
  Constant2/1 -> MinMax/2

== system c00004M_harness/Eval177 ==
  In3 : Inport
  Constant1 : Constant
  Constant2 : Constant
  Data Type Conversion2 : DataTypeConversion
  Memory3 : Memory  InitialCondition=1
  MinMax : MinMax  Inputs=3
  MinMax3 : MinMax  Inputs=2
  ROOut3 : RelationalOperator  Operator===  OutDataTypeStr=boolean  RndMeth=Simplest
  Out1 : Outport
  wires:
  Data Type Conversion2/1 -> MinMax3/1
  Memory3/1 -> MinMax3/2
  ROOut3/1 -> Data Type Conversion2/1
  MinMax3/1 -> Memory3/1, MinMax/3
  In3/1 -> ROOut3/1
  [out3] -> ROOut3/2
  MinMax/1 -> Out1/1
  Constant1/1 -> MinMax/1
  Constant2/1 -> MinMax/2

== system c00004M_harness/Eval178 ==
  In3 : Inport
  Constant1 : Constant
  Constant2 : Constant
  Data Type Conversion2 : DataTypeConversion
  Memory3 : Memory  InitialCondition=1
  MinMax : MinMax  Inputs=3
  MinMax3 : MinMax  Inputs=2
  ROOut3 : RelationalOperator  Operator===  OutDataTypeStr=boolean  RndMeth=Simplest
  Out1 : Outport
  wires:
  Data Type Conversion2/1 -> MinMax3/1
  Memory3/1 -> MinMax3/2
  ROOut3/1 -> Data Type Conversion2/1
  MinMax3/1 -> Memory3/1, MinMax/3
  In3/1 -> ROOut3/1
  [out3] -> ROOut3/2
  MinMax/1 -> Out1/1
  Constant1/1 -> MinMax/1
  Constant2/1 -> MinMax/2

== system c00004M_harness/Eval179 ==
  In3 : Inport
  Constant1 : Constant
  Constant2 : Constant
  Data Type Conversion2 : DataTypeConversion
  Memory3 : Memory  InitialCondition=1
  MinMax : MinMax  Inputs=3
  MinMax3 : MinMax  Inputs=2
  ROOut3 : RelationalOperator  Operator===  OutDataTypeStr=boolean  RndMeth=Simplest
  Out1 : Outport
  wires:
  Data Type Conversion2/1 -> MinMax3/1
  Memory3/1 -> MinMax3/2
  ROOut3/1 -> Data Type Conversion2/1
  MinMax3/1 -> Memory3/1, MinMax/3
  In3/1 -> ROOut3/1
  [out3] -> ROOut3/2
  MinMax/1 -> Out1/1
  Constant1/1 -> MinMax/1
  Constant2/1 -> MinMax/2

== system c00004M_harness/Eval180 ==
  In3 : Inport
  Constant1 : Constant
  Constant2 : Constant
  Data Type Conversion2 : DataTypeConversion
  Memory3 : Memory  InitialCondition=1
  MinMax : MinMax  Inputs=3
  MinMax3 : MinMax  Inputs=2
  ROOut3 : RelationalOperator  Operator===  OutDataTypeStr=boolean  RndMeth=Simplest
  Out1 : Outport
  wires:
  Data Type Conversion2/1 -> MinMax3/1
  Memory3/1 -> MinMax3/2
  ROOut3/1 -> Data Type Conversion2/1
  MinMax3/1 -> Memory3/1, MinMax/3
  In3/1 -> ROOut3/1
  [out3] -> ROOut3/2
  MinMax/1 -> Out1/1
  Constant1/1 -> MinMax/1
  Constant2/1 -> MinMax/2

== system c00004M_harness/Eval181 ==
  In3 : Inport
  Constant1 : Constant
  Constant2 : Constant
  Data Type Conversion2 : DataTypeConversion
  Memory3 : Memory  InitialCondition=1
  MinMax : MinMax  Inputs=3
  MinMax3 : MinMax  Inputs=2
  ROOut3 : RelationalOperator  Operator===  OutDataTypeStr=boolean  RndMeth=Simplest
  Out1 : Outport
  wires:
  Data Type Conversion2/1 -> MinMax3/1
  Memory3/1 -> MinMax3/2
  ROOut3/1 -> Data Type Conversion2/1
  MinMax3/1 -> Memory3/1, MinMax/3
  In3/1 -> ROOut3/1
  [out3] -> ROOut3/2
  MinMax/1 -> Out1/1
  Constant1/1 -> MinMax/1
  Constant2/1 -> MinMax/2

== system c00004M_harness/Eval182 ==
  In3 : Inport
  Constant1 : Constant
  Constant2 : Constant
  Data Type Conversion2 : DataTypeConversion
  Memory3 : Memory  InitialCondition=1
  MinMax : MinMax  Inputs=3
  MinMax3 : MinMax  Inputs=2
  ROOut3 : RelationalOperator  Operator===  OutDataTypeStr=boolean  RndMeth=Simplest
  Out1 : Outport
  wires:
  Data Type Conversion2/1 -> MinMax3/1
  Memory3/1 -> MinMax3/2
  ROOut3/1 -> Data Type Conversion2/1
  MinMax3/1 -> Memory3/1, MinMax/3
  In3/1 -> ROOut3/1
  [out3] -> ROOut3/2
  MinMax/1 -> Out1/1
  Constant1/1 -> MinMax/1
  Constant2/1 -> MinMax/2

== system c00004M_harness/Eval183 ==
  In3 : Inport
  Constant1 : Constant
  Constant2 : Constant
  Data Type Conversion2 : DataTypeConversion
  Memory3 : Memory  InitialCondition=1
  MinMax : MinMax  Inputs=3
  MinMax3 : MinMax  Inputs=2
  ROOut3 : RelationalOperator  Operator===  OutDataTypeStr=boolean  RndMeth=Simplest
  Out1 : Outport
  wires:
  Data Type Conversion2/1 -> MinMax3/1
  Memory3/1 -> MinMax3/2
  ROOut3/1 -> Data Type Conversion2/1
  MinMax3/1 -> Memory3/1, MinMax/3
  In3/1 -> ROOut3/1
  [out3] -> ROOut3/2
  MinMax/1 -> Out1/1
  Constant1/1 -> MinMax/1
  Constant2/1 -> MinMax/2

== system c00004M_harness/Eval184 ==
  In3 : Inport
  Constant1 : Constant
  Constant2 : Constant
  Data Type Conversion2 : DataTypeConversion
  Memory3 : Memory  InitialCondition=1
  MinMax : MinMax  Inputs=3
  MinMax3 : MinMax  Inputs=2
  ROOut3 : RelationalOperator  Operator===  OutDataTypeStr=boolean  RndMeth=Simplest
  Out1 : Outport
  wires:
  Data Type Conversion2/1 -> MinMax3/1
  Memory3/1 -> MinMax3/2
  ROOut3/1 -> Data Type Conversion2/1
  MinMax3/1 -> Memory3/1, MinMax/3
  In3/1 -> ROOut3/1
  [out3] -> ROOut3/2
  MinMax/1 -> Out1/1
  Constant1/1 -> MinMax/1
  Constant2/1 -> MinMax/2

== system c00004M_harness/Eval185 ==
  In3 : Inport
  Constant1 : Constant
  Constant2 : Constant
  Data Type Conversion2 : DataTypeConversion
  Memory3 : Memory  InitialCondition=1
  MinMax : MinMax  Inputs=3
  MinMax3 : MinMax  Inputs=2
  ROOut3 : RelationalOperator  Operator===  OutDataTypeStr=boolean  RndMeth=Simplest
  Out1 : Outport
  wires:
  Data Type Conversion2/1 -> MinMax3/1
  Memory3/1 -> MinMax3/2
  ROOut3/1 -> Data Type Conversion2/1
  MinMax3/1 -> Memory3/1, MinMax/3
  In3/1 -> ROOut3/1
  [out3] -> ROOut3/2
  MinMax/1 -> Out1/1
  Constant1/1 -> MinMax/1
  Constant2/1 -> MinMax/2

== system c00004M_harness/Eval186 ==
  In3 : Inport
  Constant1 : Constant
  Constant2 : Constant
  Data Type Conversion2 : DataTypeConversion
  Memory3 : Memory  InitialCondition=1
  MinMax : MinMax  Inputs=3
  MinMax3 : MinMax  Inputs=2
  ROOut3 : RelationalOperator  Operator===  OutDataTypeStr=boolean  RndMeth=Simplest
  Out1 : Outport
  wires:
  Data Type Conversion2/1 -> MinMax3/1
  Memory3/1 -> MinMax3/2
  ROOut3/1 -> Data Type Conversion2/1
  MinMax3/1 -> Memory3/1, MinMax/3
  In3/1 -> ROOut3/1
  [out3] -> ROOut3/2
  MinMax/1 -> Out1/1
  Constant1/1 -> MinMax/1
  Constant2/1 -> MinMax/2

== system c00004M_harness/Eval187 ==
  In3 : Inport
  Constant1 : Constant
  Constant2 : Constant
  Data Type Conversion2 : DataTypeConversion
  Memory3 : Memory  InitialCondition=1
  MinMax : MinMax  Inputs=3
  MinMax3 : MinMax  Inputs=2
  ROOut3 : RelationalOperator  Operator===  OutDataTypeStr=boolean  RndMeth=Simplest
  Out1 : Outport
  wires:
  Data Type Conversion2/1 -> MinMax3/1
  Memory3/1 -> MinMax3/2
  ROOut3/1 -> Data Type Conversion2/1
  MinMax3/1 -> Memory3/1, MinMax/3
  In3/1 -> ROOut3/1
  [out3] -> ROOut3/2
  MinMax/1 -> Out1/1
  Constant1/1 -> MinMax/1
  Constant2/1 -> MinMax/2

== system c00004M_harness/Eval188 ==
  In3 : Inport
  Constant1 : Constant
  Constant2 : Constant
  Data Type Conversion2 : DataTypeConversion
  Memory3 : Memory  InitialCondition=1
  MinMax : MinMax  Inputs=3
  MinMax3 : MinMax  Inputs=2
  ROOut3 : RelationalOperator  Operator===  OutDataTypeStr=boolean  RndMeth=Simplest
  Out1 : Outport
  wires:
  Data Type Conversion2/1 -> MinMax3/1
  Memory3/1 -> MinMax3/2
  ROOut3/1 -> Data Type Conversion2/1
  MinMax3/1 -> Memory3/1, MinMax/3
  In3/1 -> ROOut3/1
  [out3] -> ROOut3/2
  MinMax/1 -> Out1/1
  Constant1/1 -> MinMax/1
  Constant2/1 -> MinMax/2

== system c00004M_harness/Eval189 ==
  In3 : Inport
  Constant1 : Constant
  Constant2 : Constant
  Data Type Conversion2 : DataTypeConversion
  Memory3 : Memory  InitialCondition=1
  MinMax : MinMax  Inputs=3
  MinMax3 : MinMax  Inputs=2
  ROOut3 : RelationalOperator  Operator===  OutDataTypeStr=boolean  RndMeth=Simplest
  Out1 : Outport
  wires:
  Data Type Conversion2/1 -> MinMax3/1
  Memory3/1 -> MinMax3/2
  ROOut3/1 -> Data Type Conversion2/1
  MinMax3/1 -> Memory3/1, MinMax/3
  In3/1 -> ROOut3/1
  [out3] -> ROOut3/2
  MinMax/1 -> Out1/1
  Constant1/1 -> MinMax/1
  Constant2/1 -> MinMax/2

== system c00004M_harness/Eval190 ==
  In3 : Inport
  Constant1 : Constant
  Constant2 : Constant
  Data Type Conversion2 : DataTypeConversion
  Memory3 : Memory  InitialCondition=1
  MinMax : MinMax  Inputs=3
  MinMax3 : MinMax  Inputs=2
  ROOut3 : RelationalOperator  Operator===  OutDataTypeStr=boolean  RndMeth=Simplest
  Out1 : Outport
  wires:
  Data Type Conversion2/1 -> MinMax3/1
  Memory3/1 -> MinMax3/2
  ROOut3/1 -> Data Type Conversion2/1
  MinMax3/1 -> Memory3/1, MinMax/3
  In3/1 -> ROOut3/1
  [out3] -> ROOut3/2
  MinMax/1 -> Out1/1
  Constant1/1 -> MinMax/1
  Constant2/1 -> MinMax/2

== system c00004M_harness/Eval191 ==
  In3 : Inport
  Constant1 : Constant
  Constant2 : Constant
  Data Type Conversion2 : DataTypeConversion
  Memory3 : Memory  InitialCondition=1
  MinMax : MinMax  Inputs=3
  MinMax3 : MinMax  Inputs=2
  ROOut3 : RelationalOperator  Operator===  OutDataTypeStr=boolean  RndMeth=Simplest
  Out1 : Outport
  wires:
  Data Type Conversion2/1 -> MinMax3/1
  Memory3/1 -> MinMax3/2
  ROOut3/1 -> Data Type Conversion2/1
  MinMax3/1 -> Memory3/1, MinMax/3
  In3/1 -> ROOut3/1
  [out3] -> ROOut3/2
  MinMax/1 -> Out1/1
  Constant1/1 -> MinMax/1
  Constant2/1 -> MinMax/2

== system c00004M_harness/Eval192 ==
  In3 : Inport
  Constant1 : Constant
  Constant2 : Constant
  Data Type Conversion2 : DataTypeConversion
  Memory3 : Memory  InitialCondition=1
  MinMax : MinMax  Inputs=3
  MinMax3 : MinMax  Inputs=2
  ROOut3 : RelationalOperator  Operator===  OutDataTypeStr=boolean  RndMeth=Simplest
  Out1 : Outport
  wires:
  Data Type Conversion2/1 -> MinMax3/1
  Memory3/1 -> MinMax3/2
  ROOut3/1 -> Data Type Conversion2/1
  MinMax3/1 -> Memory3/1, MinMax/3
  In3/1 -> ROOut3/1
  [out3] -> ROOut3/2
  MinMax/1 -> Out1/1
  Constant1/1 -> MinMax/1
  Constant2/1 -> MinMax/2

== system c00004M_harness/Eval193 ==
  In3 : Inport
  Constant1 : Constant
  Constant2 : Constant
  Data Type Conversion2 : DataTypeConversion
  Memory3 : Memory  InitialCondition=1
  MinMax : MinMax  Inputs=3
  MinMax3 : MinMax  Inputs=2
  ROOut3 : RelationalOperator  Operator===  OutDataTypeStr=boolean  RndMeth=Simplest
  Out1 : Outport
  wires:
  Data Type Conversion2/1 -> MinMax3/1
  Memory3/1 -> MinMax3/2
  ROOut3/1 -> Data Type Conversion2/1
  MinMax3/1 -> Memory3/1, MinMax/3
  In3/1 -> ROOut3/1
  [out3] -> ROOut3/2
  MinMax/1 -> Out1/1
  Constant1/1 -> MinMax/1
  Constant2/1 -> MinMax/2

== system c00004M_harness/Eval194 ==
  In3 : Inport
  Constant1 : Constant
  Constant2 : Constant
  Data Type Conversion2 : DataTypeConversion
  Memory3 : Memory  InitialCondition=1
  MinMax : MinMax  Inputs=3
  MinMax3 : MinMax  Inputs=2
  ROOut3 : RelationalOperator  Operator===  OutDataTypeStr=boolean  RndMeth=Simplest
  Out1 : Outport
  wires:
  Data Type Conversion2/1 -> MinMax3/1
  Memory3/1 -> MinMax3/2
  ROOut3/1 -> Data Type Conversion2/1
  MinMax3/1 -> Memory3/1, MinMax/3
  In3/1 -> ROOut3/1
  [out3] -> ROOut3/2
  MinMax/1 -> Out1/1
  Constant1/1 -> MinMax/1
  Constant2/1 -> MinMax/2

== system c00004M_harness/Eval195 ==
  In3 : Inport
  Constant1 : Constant
  Constant2 : Constant
  Data Type Conversion2 : DataTypeConversion
  Memory3 : Memory  InitialCondition=1
  MinMax : MinMax  Inputs=3
  MinMax3 : MinMax  Inputs=2
  ROOut3 : RelationalOperator  Operator===  OutDataTypeStr=boolean  RndMeth=Simplest
  Out1 : Outport
  wires:
  Data Type Conversion2/1 -> MinMax3/1
  Memory3/1 -> MinMax3/2
  ROOut3/1 -> Data Type Conversion2/1
  MinMax3/1 -> Memory3/1, MinMax/3
  In3/1 -> ROOut3/1
  [out3] -> ROOut3/2
  MinMax/1 -> Out1/1
  Constant1/1 -> MinMax/1
  Constant2/1 -> MinMax/2

== system c00004M_harness/Eval196 ==
  In3 : Inport
  Constant1 : Constant
  Constant2 : Constant
  Data Type Conversion2 : DataTypeConversion
  Memory3 : Memory  InitialCondition=1
  MinMax : MinMax  Inputs=3
  MinMax3 : MinMax  Inputs=2
  ROOut3 : RelationalOperator  Operator===  OutDataTypeStr=boolean  RndMeth=Simplest
  Out1 : Outport
  wires:
  Data Type Conversion2/1 -> MinMax3/1
  Memory3/1 -> MinMax3/2
  ROOut3/1 -> Data Type Conversion2/1
  MinMax3/1 -> Memory3/1, MinMax/3
  In3/1 -> ROOut3/1
  [out3] -> ROOut3/2
  MinMax/1 -> Out1/1
  Constant1/1 -> MinMax/1
  Constant2/1 -> MinMax/2

== system c00004M_harness/Eval197 ==
  In3 : Inport
  Constant1 : Constant
  Constant2 : Constant
  Data Type Conversion2 : DataTypeConversion
  Memory3 : Memory  InitialCondition=1
  MinMax : MinMax  Inputs=3
  MinMax3 : MinMax  Inputs=2
  ROOut3 : RelationalOperator  Operator===  OutDataTypeStr=boolean  RndMeth=Simplest
  Out1 : Outport
  wires:
  Data Type Conversion2/1 -> MinMax3/1
  Memory3/1 -> MinMax3/2
  ROOut3/1 -> Data Type Conversion2/1
  MinMax3/1 -> Memory3/1, MinMax/3
  In3/1 -> ROOut3/1
  [out3] -> ROOut3/2
  MinMax/1 -> Out1/1
  Constant1/1 -> MinMax/1
  Constant2/1 -> MinMax/2

== system c00004M_harness/Eval198 ==
  In3 : Inport
  Constant1 : Constant
  Constant2 : Constant
  Data Type Conversion2 : DataTypeConversion
  Memory3 : Memory  InitialCondition=1
  MinMax : MinMax  Inputs=3
  MinMax3 : MinMax  Inputs=2
  ROOut3 : RelationalOperator  Operator===  OutDataTypeStr=boolean  RndMeth=Simplest
  Out1 : Outport
  wires:
  Data Type Conversion2/1 -> MinMax3/1
  Memory3/1 -> MinMax3/2
  ROOut3/1 -> Data Type Conversion2/1
  MinMax3/1 -> Memory3/1, MinMax/3
  In3/1 -> ROOut3/1
  [out3] -> ROOut3/2
  MinMax/1 -> Out1/1
  Constant1/1 -> MinMax/1
  Constant2/1 -> MinMax/2

== system c00004M_harness/Eval199 ==
  In3 : Inport
  Constant1 : Constant
  Constant2 : Constant
  Data Type Conversion2 : DataTypeConversion
  Memory3 : Memory  InitialCondition=1
  MinMax : MinMax  Inputs=3
  MinMax3 : MinMax  Inputs=2
  ROOut3 : RelationalOperator  Operator===  OutDataTypeStr=boolean  RndMeth=Simplest
  Out1 : Outport
  wires:
  Data Type Conversion2/1 -> MinMax3/1
  Memory3/1 -> MinMax3/2
  ROOut3/1 -> Data Type Conversion2/1
  MinMax3/1 -> Memory3/1, MinMax/3
  In3/1 -> ROOut3/1
  [out3] -> ROOut3/2
  MinMax/1 -> Out1/1
  Constant1/1 -> MinMax/1
  Constant2/1 -> MinMax/2

== system c00004M_harness/Eval200 ==
  In3 : Inport
  Constant1 : Constant
  Constant2 : Constant
  Data Type Conversion2 : DataTypeConversion
  Memory3 : Memory  InitialCondition=1
  MinMax : MinMax  Inputs=3
  MinMax3 : MinMax  Inputs=2
  ROOut3 : RelationalOperator  Operator===  OutDataTypeStr=boolean  RndMeth=Simplest
  Out1 : Outport
  wires:
  Data Type Conversion2/1 -> MinMax3/1
  Memory3/1 -> MinMax3/2
  ROOut3/1 -> Data Type Conversion2/1
  MinMax3/1 -> Memory3/1, MinMax/3
  In3/1 -> ROOut3/1
  [out3] -> ROOut3/2
  MinMax/1 -> Out1/1
  Constant1/1 -> MinMax/1
  Constant2/1 -> MinMax/2
